simulink model "LQR_sim"  (R2022b)
settings: Solver=FixedStepAuto  StartTime=0.0  StopTime=30  RelTol=1e-3
values from neighbouring files (symbols this model uses):
  A = [0    -g   0    0    0    0    0    0 ... (first row only)    [LQR_fiveDOF.m]
  B = [0          g       0       0 ... (first row only)    [LQR_fiveDOF.m]
  C = eye(8)    [LQR_fiveDOF.m]
  g = 9.82    [LQR_fiveDOF.m]
undefined symbols (not defined in the file or in its folder): DiscIntNeverNeededParam, Kd
settings Model: Creator=Edvin  LastModifiedBy=Edvin
settings OptimizationCC: OptimizeBlockIOStorage=off  ZeroExternalMemoryAtStartup=off  ZeroInternalMemoryAtStartup=off  OptimizeDataStoreBuffers=off  BusAssignmentInplaceUpdate=off
settings DebuggingCC: SFUnexpectedBacktrackingDiag=warning  SFNoUnconditionalDefaultTransitionDiag=warning
settings HardwareCC: ProdBitPerPointer=32  ProdBitPerSizeT=32  ProdBitPerPtrDiffT=32  ProdLargestAtomicInteger=Long  ProdLargestAtomicFloat=Double  ProdWordSize=32  ProdHWDeviceType=ARM Compatible->ARM Cortex-M
settings RTWCC: GenCodeOnly=on  GenerateReport=on  Toolchain=Microsoft Visual C++ 2022 v17.0 | nmake (64-bit Windows)  BuildConfiguration=Debug  LaunchReport=on  TargetLang=C++
settings CodeAppCC: ForceParamTrailComments=on  MATLABSourceComments=on  EnableCustomComments=on
settings GRTTargetCC: TargetLangStandard=C++11 (ISO)  CombineSignalStateStructs=on  CodeInterfacePackaging=C++ class  SupportVariableSizeSignals=on  MultiInstanceErrorCode=Warning

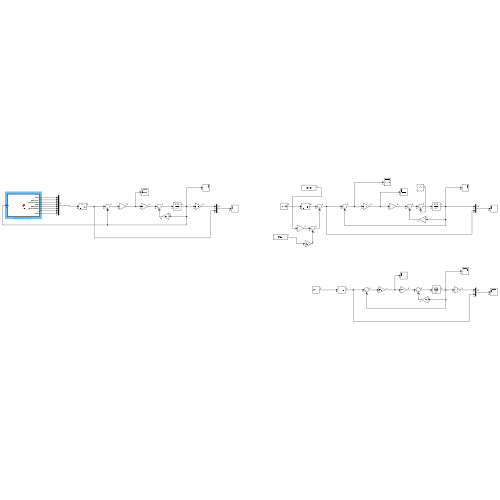
[thumbnail: Simulink's stored preview of the top-level diagram]
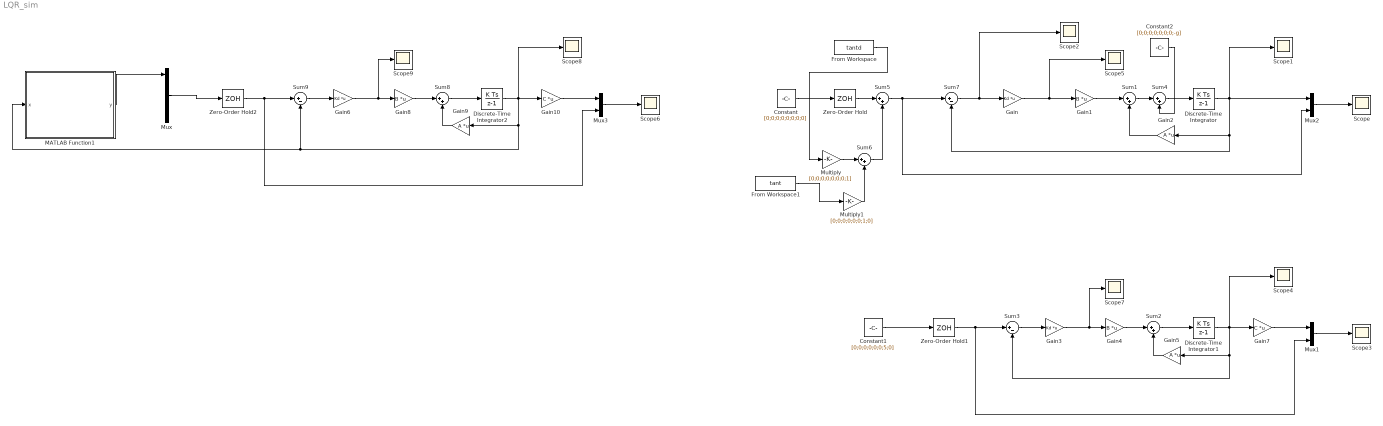
== system LQR_sim ==
  Constant : Constant  Value=[0;0;0;0;0;0;0;0]
  Constant1 : Constant  Value=[0;0;0;0;0;0;5;0]
  Constant2 : Constant  Value=[0;0;0;0;0;0;0;-g]
  Discrete-Time Integrator : DiscreteIntegrator  SampleTime=-1  ICPrevOutput=DiscIntNeverNeededParam  ICPrevScaledInput=DiscIntNeverNeededParam
  Discrete-Time Integrator1 : DiscreteIntegrator  SampleTime=-1  ICPrevOutput=DiscIntNeverNeededParam  ICPrevScaledInput=DiscIntNeverNeededParam
  Discrete-Time Integrator2 : DiscreteIntegrator  SampleTime=-1  ICPrevOutput=DiscIntNeverNeededParam  ICPrevScaledInput=DiscIntNeverNeededParam
  From Workspace : FromWorkspace  VariableName=tantd  SampleTime=0.01
  From Workspace1 : FromWorkspace  VariableName=tant
  Gain : Gain  Gain=Kd  Multiplication=Matrix(K*u)
  Gain1 : Gain  Gain=B  Multiplication=Matrix(K*u)
  Gain10 : Gain  Gain=C  Multiplication=Matrix(K*u)
  Gain2 : Gain  Gain=A  Multiplication=Matrix(K*u)
  Gain3 : Gain  Gain=Kd  Multiplication=Matrix(K*u)
  Gain4 : Gain  Gain=B  Multiplication=Matrix(K*u)
  Gain5 : Gain  Gain=A  Multiplication=Matrix(K*u)
  Gain6 : Gain  Gain=Kd  Multiplication=Matrix(K*u)
  Gain7 : Gain  Gain=C  Multiplication=Matrix(K*u)
  Gain8 : Gain  Gain=B  Multiplication=Matrix(K*u)
  Gain9 : Gain  Gain=A  Multiplication=Matrix(K*u)
  MATLAB Function1 : MATLAB Function  TreatAsAtomicUnit=on
  Multiply : Gain  Gain=[0;0;0;0;0;0;0;1]
  Multiply1 : Gain  Gain=[0;0;0;0;0;0;1;0]
  Mux : Mux  Inputs=8
  Mux1 : Mux  Inputs=2
  Mux2 : Mux  Inputs=2
  Mux3 : Mux  Inputs=2
  Scope{,1..9} (10 alike) : Scope
  Sum{1..2,4..6,8} (6 alike) : Sum  Inputs=|++
  Sum3 : Sum  Inputs=|+-
  Sum7 : Sum  Inputs=|+-
  Sum9 : Sum  Inputs=|+-
  Zero-Order Hold : ZeroOrderHold  SampleTime=0.01
  Zero-Order Hold1 : ZeroOrderHold  SampleTime=0.01
  Zero-Order Hold2 : ZeroOrderHold  SampleTime=0.01
  wires:
  Gain1/1 -> Sum1/1
  Gain2/1 -> Sum1/2
  Constant/1 -> Zero-Order Hold/1
  Mux2/1 -> Scope/1
  Discrete-Time Integrator/1 -> Gain2/1, Sum7/2, Scope1/1, Mux2/1
  Sum7/1 -> Gain/1, Scope2/1
  Sum2/1 -> Discrete-Time Integrator1/1
  Gain4/1 -> Sum2/1
  Mux1/1 -> Scope3/1
  Zero-Order Hold1/1 -> Sum3/1, Mux1/2
  Constant1/1 -> Zero-Order Hold1/1
  Discrete-Time Integrator1/1 -> Gain7/1, Scope4/1, Sum3/2, Gain5/1
  Gain5/1 -> Sum2/2
  Gain7/1 -> Mux1/1
  Gain3/1 -> Scope7/1, Gain4/1
  Sum3/1 -> Gain3/1
  Gain/1 -> Gain1/1, Scope5/1
  Sum4/1 -> Discrete-Time Integrator/1
  Sum1/1 -> Sum4/1
  Constant2/1 -> Sum4/2
  Zero-Order Hold/1 -> Sum5/1
  Sum5/1 -> Mux2/2, Sum7/1
  From Workspace/1 -> Multiply/1
  Multiply/1 -> Sum6/1
  Sum6/1 -> Sum5/2
  Multiply1/1 -> Sum6/2
  From Workspace1/1 -> Multiply1/1
  Gain9/1 -> Sum8/2
  Discrete-Time Integrator2/1 -> Gain10/1, Scope8/1, Sum9/2, MATLAB Function1/1(x), Gain9/1
  Gain8/1 -> Sum8/1
  Zero-Order Hold2/1 -> Sum9/1, Mux3/2
  Mux3/1 -> Scope6/1
  Gain10/1 -> Mux3/1
  Sum8/1 -> Discrete-Time Integrator2/1
  Sum9/1 -> Gain6/1
  Gain6/1 -> Scope9/1, Gain8/1
  Mux/1 -> Zero-Order Hold2/1
  MATLAB Function1/1(y) -> Mux/1
  ? -> Mux/2
  ? -> Mux/3
  ? -> Mux/4
  ? -> Mux/5
  ? -> Mux/6
  ? -> Mux/7
  ? -> Mux/8

== matlab function LQR_sim/MATLAB Function1 ==
  data: x input; y output
function y = fcn(x)
% initial defenitions:
fmax = 3;

% set desired references for final position
xdotref = 0;
gamma1ref = 0;
gamma1dotref = 0;
ydotref = 0;
gamma2ref = 0;
gamma2dotref = 0;
zref = 3;
zdotref = 0;

% extract altitude and velocity and calculate the error
zpos = x(7);
zdotvel = x(8);
zerror = zref - zpos;
%velerror = zdotref - zdotvel;

zoutput = 0;
zdotoutput = 0;
if zerror ~= 0   %check if there is an error
    zoutput = 0.001*zerror;

    if alterror/zref > 0.5  %check if the half way point is reached, based on this increase or decrease the velocity reference
        zdotoutput = zdotvel + 0.01*fmax;
    else
        zdotoutput = zdotvel - 0.01*fmax;
    end
    
end

y = [xdot; gamma1; gamma1dot; ydot; gamma2; gamma2dot; zoutput; zdotoutput ];
